simulink model "Autopilot_Simulator"  (R2022a)
settings: Solver=ode4  StartTime=0.0  StopTime=1500  FixedStep=0.01  RelTol=1e-3
model workspace: external: MAT-File C:\Users\kkshu\Desktop\GNC MQ9_Autopilot Final\Simulink\MQ9_reaper_drone.mat (data not in the file)
values from neighbouring files (symbols this model uses):
  p_0 = 0    [MQ9_reaper_drone.mat]    (also in ReadExcelModified.m = s0(4))
  phi_0 = 0    [MQ9_reaper_drone.mat]    (also in ReadExcelModified.m = s0(7))
  psi_0 = 0    [MQ9_reaper_drone.mat]    (also in ReadExcelModified.m = s0(9))
  q_0 = 0    [MQ9_reaper_drone.mat]    (also in ReadExcelModified.m = s0(5))
  r_0 = 0    [MQ9_reaper_drone.mat]    (also in ReadExcelModified.m = s0(6))
  theta_0 = 0.0471238898038    [MQ9_reaper_drone.mat]    (also in ReadExcelModified.m = s0(8))
  u_0 = 585.349466728    [MQ9_reaper_drone.mat]    (also in ReadExcelModified.m = s0(1))
  v_0 = 0    [MQ9_reaper_drone.mat]    (also in ReadExcelModified.m = s0(2))
  Vto = 586    [MQ9_reaper_drone.mat]    (also in ReadExcelModified.m = sqrt(s0(1)^2 + s0(2)^2 + s0(3)^2))
  w_0 = 27.6043801159    [MQ9_reaper_drone.mat]    (also in ReadExcelModified.m = s0(3))
  x_0 = 0    [MQ9_reaper_drone.mat]    (also in ReadExcelModified.m = s0(10))
  y_0 = 0    [MQ9_reaper_drone.mat]    (also in ReadExcelModified.m = s0(11))
  z_0 = 0    [MQ9_reaper_drone.mat]    (also in ReadExcelModified.m = s0(12))
undefined symbols (not defined in the file or in its folder): Earth, JSBSim2, MQ, sigbuilder_block, WGS84
libraries: simulink_extras x3, aerolibfltsims x2, aerolibtransform2 x1
settings Model: PacingRate=22  Creator=mohan  LastModifiedBy=kkshu
settings SolverCC: AlgebraicLoopSolver=TrustRegion
settings DebuggingCC: UnconnectedInputMsg=warning  UnconnectedOutputMsg=warning  UnconnectedLineMsg=warning  SFMachineParentedDataDiag=warning

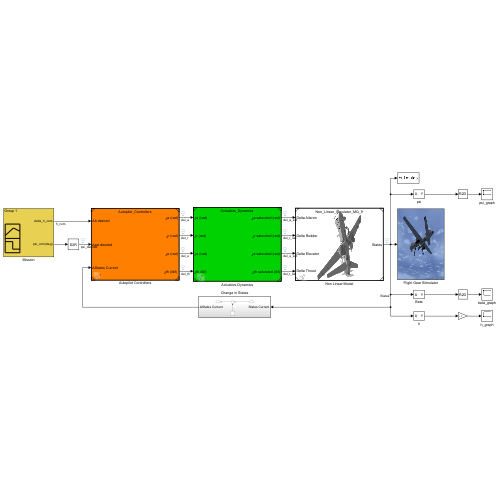
[thumbnail: Simulink's stored preview of the top-level diagram]
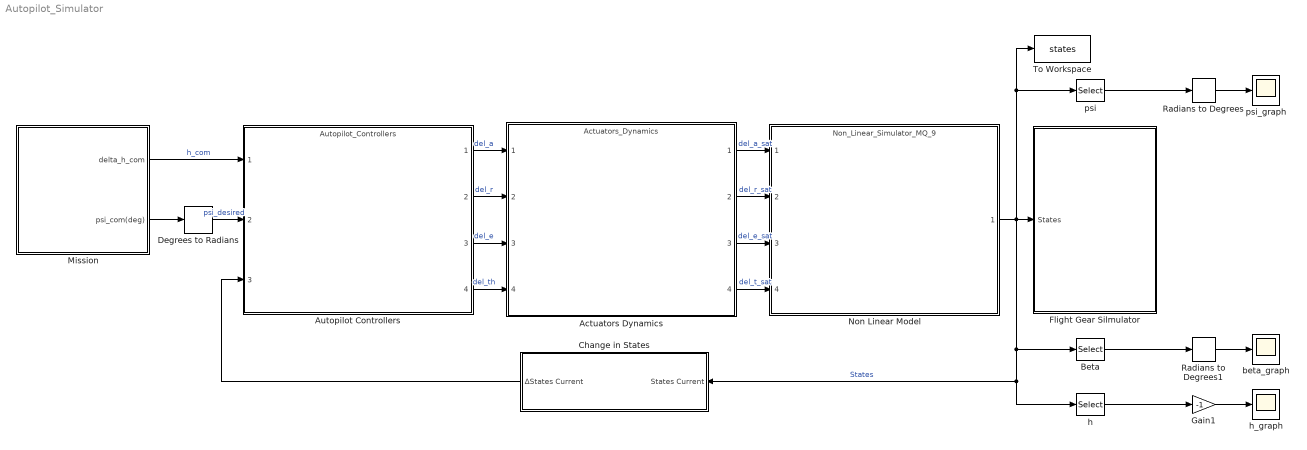
== system Autopilot_Simulator ==
  Actuators Dynamics : ModelReference  ModelNameDialog=Actuators_Dynamics.slx  SimulationMode=Normal  ModelReferenceVersion=5.3
  Autopilot Controllers : ModelReference  ModelNameDialog=Autopilot_Controllers.slx  SimulationMode=Normal  ModelReferenceVersion=5.6
  Beta : Selector  InputPortWidth=15  IndexOptions=Index vector (dialog)  Indices=14  OutputSizes=1
  Change in States : Subsystem
  Degrees to Radians : simulink_extras/Transformations/Degrees to Radians
  Flight Gear Silmulator : Subsystem
      mask Display: image('C:\Users\kkshu\Desktop\GNC PPT\GNC MQ9 Image\flightgear2.jpg'); % Use "Edit Image" on toolstrip to change.
  Gain1 : Gain  Gain=-1
  Mission : Subsystem  Tag=STV Subsys  LoadFcn=sigbuilder_block('load');  StartFcn=sigbuilder_block('start');  StopFcn=sigbuilder_block('stop');  ClipboardFcn=sigbuilder_block('clipboard');  mask(Sigbuilder block){tuvar=[0:10]}
      mask help: Simulink:masks:SigbuilderBlock_MD
      mask init:
      | if ~strcmp(get_param(bdroot(gcbh),'SimulationStatus'),'stopped') tuvar = sigbuilder_block('maskInit'); end
      settings: CopyFcn=sigbuilder_block('copy');  DeleteFcn=sigbuilder_block('delete');  ModelCloseFcn=sigbuilder_block('modelClose');  PreSaveFcn=sigbuilder_block('preSave');  PauseFcn=sigbuilder_block('pause');  ContinueFcn=sigbuilder_block('continue');  NameChangeFcn=sigbuilder_block('namechange');  OpenFcn=sigbuilder_block('open',[265.5 96 689 362.5 ]);  CloseFcn=sigbuilder_block('close');
      mask Display: plot(0, 0, 100, 100,[2, 2, 32, 32, 2], [68, 8, 8, 68, 68],[32, 2], [38, 38], [32, 19, 2],[53, 60, 44], [32, 17, 17, 2],[16, 16, 31, 31]);txt = getActiveGroup(gcbh);text(2, 100, txt,'verticalAlignment', 'top');
  Non Linear Model : ModelReference  ModelNameDialog=Non_Linear_Simulator_MQ_9.slx  SimulationMode=Normal  ModelReferenceVersion=5.2
      mask Display: image('$imagefile'); % Use "Edit Image" on toolstrip to change.
  Radians to Degrees : simulink_extras/Transformations/Radians to Degrees
  Radians to Degrees1 : simulink_extras/Transformations/Radians to Degrees
  To Workspace : ToWorkspace  VariableName=states  SaveFormat=Timeseries  SampleTime=-1
  beta_graph : Scope
  h : Selector  InputPortWidth=15  IndexOptions=Index vector (dialog)  Indices=3  OutputSizes=1
  h_graph : Scope
  psi : Selector  InputPortWidth=15  IndexOptions=Index vector (dialog)  Indices=6  OutputSizes=1
  psi_graph : Scope
  wires:
  Beta/1 -> Radians to Degrees1/1
  Radians to Degrees/1 -> psi_graph/1
  Gain1/1 -> h_graph/1
  psi/1 -> Radians to Degrees/1
  Change in States/1(ΔStates Current) -> Autopilot Controllers/3
  h/1 -> Gain1/1
  Radians to Degrees1/1 -> beta_graph/1
  Degrees to Radians/1 -> Autopilot Controllers/2  "psi_desired"
  Mission/1(delta_h_com) -> Autopilot Controllers/1  "h_com"
  Mission/2(psi_com(deg)) -> Degrees to Radians/1
  Autopilot Controllers/4 -> Actuators Dynamics/4  "del_th"
  Autopilot Controllers/3 -> Actuators Dynamics/3  "del_e"
  Autopilot Controllers/2 -> Actuators Dynamics/2  "del_r"
  Autopilot Controllers/1 -> Actuators Dynamics/1  "del_a"
  Actuators Dynamics/4 -> Non Linear Model/4  "del_t_sat"
  Actuators Dynamics/3 -> Non Linear Model/3  "del_e_sat"
  Actuators Dynamics/2 -> Non Linear Model/2  "del_r_sat"
  Actuators Dynamics/1 -> Non Linear Model/1  "del_a_sat"
  Non Linear Model/1 -> h/1, Change in States/1(States Current), Beta/1, psi/1, To Workspace/1, Flight Gear Silmulator/1(States)  "States"

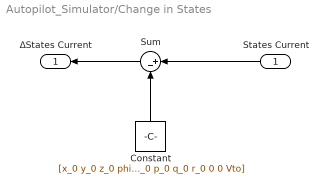
== system Autopilot_Simulator/Change in States ==
  States Current : Inport
  Constant : Constant  Value=[x_0 y_0 z_0 phi_0 theta_0 psi_0 u_0 v_0 w_0 p_0 q_0 r_0 0 0 Vto]
  Sum : Sum  Inputs=|+-
  ΔStates Current : Outport
  wires:
  States Current/1 -> Sum/1
  Constant/1 -> Sum/2
  Sum/1 -> ΔStates Current/1

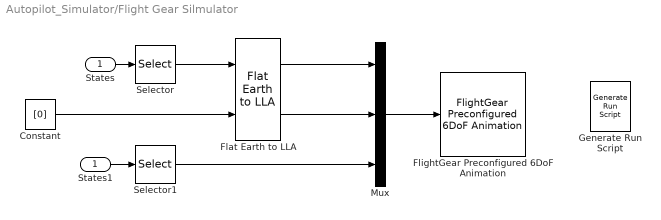
== system Autopilot_Simulator/Flight Gear Silmulator ==
  States : Inport
  Constant : Constant  Value=[0]
  Flat Earth to LLA : aerolibtransform2/Flat Earth to LLA  units=Metric (MKS)  ptype=Earth (WGS84)  F=1/298.257223563  R=6378137  refPosPort=off  LL0=[0 10]  psi=0
  FlightGear Preconfigured 6DoF Animation : aerolibfltsims/FlightGear Preconfigured 6DoF Animation  xFlightGearVersion=v2019.1  DestinationIpAddress=127.0.0.1  DestinationPort=5502  SampleTime=-1  packetVersion=24
  Generate Run Script : aerolibfltsims/Generate Run Script  Architecture=Win64  dataFlow=Send  GeometryModelName=MQ-9-JSBSim2  AirportId=PHTO  RunwayId=08  InitialAltitude=7224  InitialHeading=0  OffsetDistance=0  OffsetAzimuth=0  InstallScenery=on  DisableShaders=off  OriginAddress=127.0.0.1  DestinationPort=5502  OriginPort=5505  LocalAddress=127.0.0.1  OutputFileName=runfg.bat  FlightGearBaseDirectory=C:\Program Files\FlightGear
  Mux : Mux  Inputs=3
  Selector : Selector  InputPortWidth=15  IndexOptions=Index vector (dialog)  Indices=[1 2 3]  OutputSizes=1
  Selector1 : Selector  InputPortWidth=15  IndexOptions=Index vector (dialog)  Indices=[4 5 6]  OutputSizes=1
  States1 : InportShadow
  wires:
  Flat Earth to LLA/1 -> Mux/1
  Selector/1 -> Flat Earth to LLA/1
  Flat Earth to LLA/2 -> Mux/2
  States/1 -> Selector/1
  States1/1 -> Selector1/1
  Selector1/1 -> Mux/3
  Mux/1 -> FlightGear Preconfigured 6DoF Animation/1
  Constant/1 -> Flat Earth to LLA/2

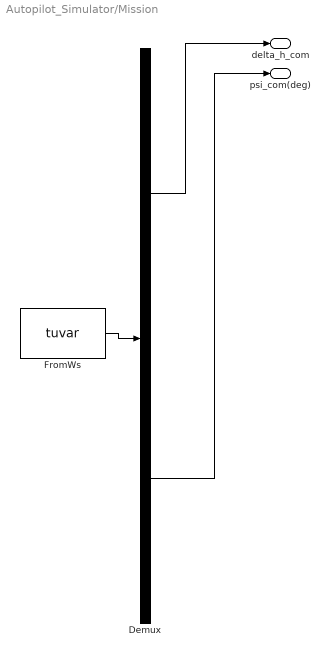
== system Autopilot_Simulator/Mission ==
  Demux : Demux  Tag=STV Demux  Outputs=2
      settings: DisplayOption=none
  FromWs : FromWorkspace  Tag=STV FromWs  VariableName=tuvar
      SigBuilderData=|
      | common.afterFinalStr = 'Extrapolate'
      | common.sampleTime = 0
      | dataSet.timeRange = [0 1500]
      | dataSet.name = 'Group 1'
      | sbobj.Groups.Name = 'Group 1'
      | sbobj.Groups.Signals(1).Name = 'delta_h_com'
      | sbobj.Groups.Signals(1).XData = [0 400.2 940.2 940.2 1060.2 1460.4 1500]
      | sbobj.Groups.Signals(1).YData = [0 10000 10000 10100 10100 10.0949525237 10.0949525237]
      | sbobj.Groups.Signals(2).Name = 'psi_com(deg)'
      | sbobj.Groups.Signals(2).XData = [0 510 510 700 700 1500]
      | sbobj.Groups.Signals(2).YData = [0 0 360 360 0 0]
      | sbobj.Groups.TimeRange = [0 1500]
  delta_h_com : Outport  Tag=STV Outport
  psi_com(deg) : Outport  Tag=STV Outport  Port=2
  wires:
  Demux/1 -> delta_h_com/1
  FromWs/1 -> Demux/1
  Demux/2 -> psi_com(deg)/1
